simulink model "p1b2"  (R2023b)
settings: Solver=VariableStepAuto  StartTime=0.0  StopTime=75  RelTol=1e-3
settings Model: Creator=tanvi  LastModifiedBy=tanvi

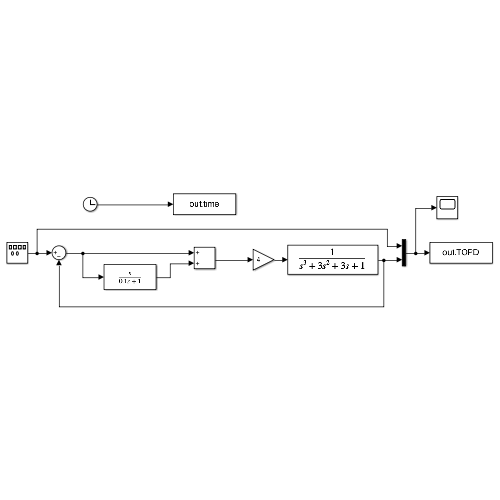
[thumbnail: Simulink's stored preview of the top-level diagram]
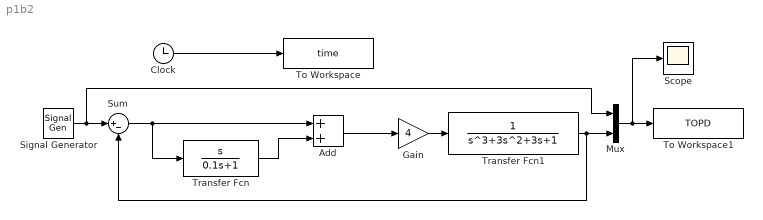
== system p1b2 ==
  Add : Sum
  Clock : Clock
  Gain : Gain  Gain=4
  Mux : Mux  Inputs=2
  Scope : Scope
  Signal Generator : SignalGenerator  WaveForm=square  Frequency=0.02
  Sum : Sum  Inputs=|+-
  To Workspace : ToWorkspace  VariableName=time  SampleTime=-1
  To Workspace1 : ToWorkspace  VariableName=TOPD  SampleTime=-1
  Transfer Fcn : TransferFcn  Numerator=[1 0]  Denominator=[0.1 1]
  Transfer Fcn1 : TransferFcn  Denominator=[1 3 3 1]
  wires:
  Transfer Fcn/1 -> Add/2
  Signal Generator/1 -> Mux/1, Sum/1
  Sum/1 -> Transfer Fcn/1, Add/1
  Transfer Fcn1/1 -> Sum/2, Mux/2
  Add/1 -> Gain/1
  Gain/1 -> Transfer Fcn1/1
  Mux/1 -> Scope/1, To Workspace1/1
  Clock/1 -> To Workspace/1
